simulink model "ThreePhasePVModule"  (R2025b)
settings: Solver=VariableStepAuto  StartTime=0.0  StopTime=1  RelTol=1e-3
undefined symbols (not defined in the file): Ppv
libraries: fl_lib x7, nesl_utility x5, simulink x1
settings Model: Creator=a6039  LastModifiedBy=agarcian
settings SolverCC: AlgebraicLoopSolver=TrustRegion
settings DebuggingCC: UnconnectedInputMsg=warning  UnconnectedOutputMsg=warning  UnconnectedLineMsg=warning
settings ModelReferenceCC: EnableRefExpFcnMdlSchedulingChecks=on
settings RTWCC: GPUComputeCapability=3.5  DLArmComputeVersion=19.05

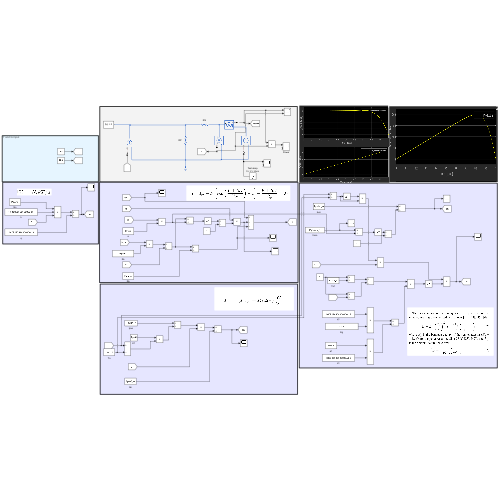
[thumbnail: Simulink's stored preview of the top-level diagram]
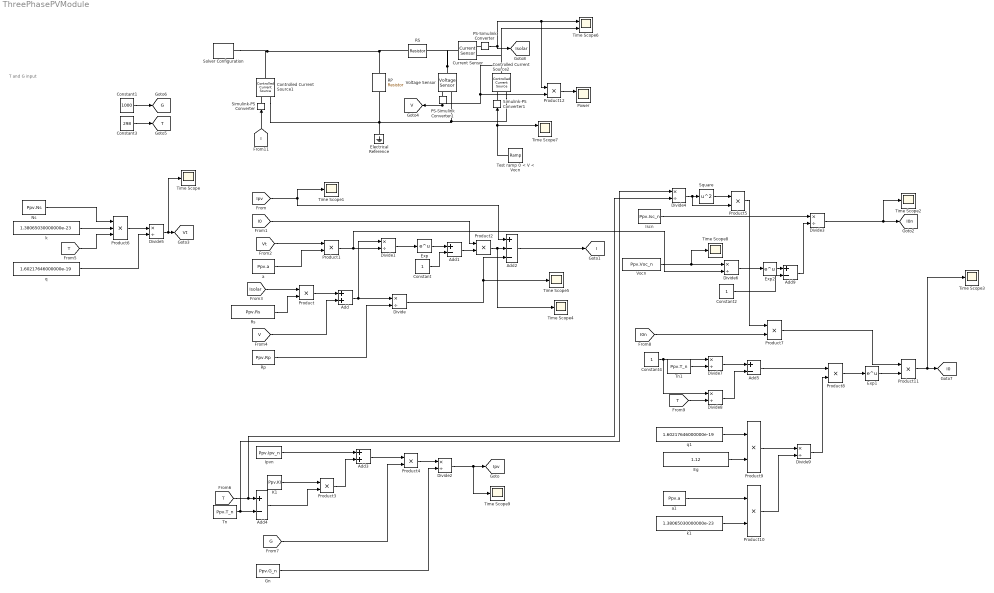
== system ThreePhasePVModule ==
  note: T and G input
  Add : Sum
  Add{1,4..5,9} (4 alike) : Sum  Inputs=+-
  Add2 : Sum  Inputs=+--
  Add3 : Sum
  Constant : Constant
  Constant1 : Constant  Value=1000
  Constant2 : Constant
  Constant3 : Constant  Value=298
  Constant4 : Constant
  Controlled Current Source1 : fl_lib/Electrical/Electrical Sources/Controlled Current Source
  Controlled Current Source2 : fl_lib/Electrical/Electrical Sources/Controlled Current Source
  Current Sensor : fl_lib/Electrical/Electrical Sensors/Current Sensor
  Divide{,1..9} (10 alike) : Product  Inputs=*/
  Eg : Constant  Value=1.12
  Electrical Reference : fl_lib/Electrical/Electrical Elements/Electrical Reference
  Exp : Math
  Exp1 : Math
  Exp2 : Math
  Gn : Constant  Value=Ppv.G_n
  Ipvn : Constant  Value=Ppv.Ipv_n
  Iscn : Constant  Value=Ppv.Isc_n
  K1 : Constant  Value=Ppv.KI
  Ns : Constant  Value=Ppv.Ns
  PS-Simulink Converter : nesl_utility/PS-Simulink Converter  PhysicalDomain=network_engine_domain  SubClassName=ps_output  LeftPortType=input  RightPortType=output  PseudoPeriodic=off  Frequencies=[]  VectorFormat=inherit  Unit=inherit  AffineConversion=off
  PS-Simulink Converter1 : nesl_utility/PS-Simulink Converter  PhysicalDomain=network_engine_domain  SubClassName=ps_output  LeftPortType=input  RightPortType=output  PseudoPeriodic=off  Frequencies=[]  VectorFormat=inherit  Unit=inherit  AffineConversion=off
  Power : Scope  NumInputPorts=2
      settings: TimeUnits=Metric (based on Time Span)  ActiveDisplayYMinimum=-158.2887  ActiveDisplayYMaximum=34.79764  YLabel=Amplitude  DataLoggingVariableName=ScopeData9
  Product{,1..5,7..12} (12 alike) : Product
  Product6 : Product  Inputs=3
  RP : fl_lib/Electrical/Electrical Elements/Resistor  R=Ppv.Rp Ohm  i_specify=off  i_priority=None  i=0 A  i_nominal_specify=off  i_nominal_value=1  i_nominal_unit=A  v_specify=off  v_priority=None  v=0 V  v_nominal_specify=off  v_nominal_value=1  v_nominal_unit=V
  RS : fl_lib/Electrical/Electrical Elements/Resistor  R=Ppv.Rs Ohm  i_specify=off  i_priority=None  i=0 A  i_nominal_specify=off  i_nominal_value=1  i_nominal_unit=A  v_specify=off  v_priority=None  v=0 V  v_nominal_specify=off  v_nominal_value=1  v_nominal_unit=V
  Rp : Constant  Value=Ppv.Rp
  Rs : Constant  Value=Ppv.Rs
  Simulink-PS Converter : nesl_utility/Simulink-PS Converter  PhysicalDomain=network_engine_domain  SubClassName=ps_input  LeftPortType=input  RightPortType=output  PseudoPeriodic=off  Frequencies=[]  NoiseDistribution=none  NoiseParameters=[]  Unit=1  AffineConversion=off  FilteringAndDerivatives=provide  SimscapeFilterOrder=1  InputFilterTimeConstant=0.001  UdotUserProvided=0
  Simulink-PS Converter1 : nesl_utility/Simulink-PS Converter  PhysicalDomain=network_engine_domain  SubClassName=ps_input  LeftPortType=input  RightPortType=output  PseudoPeriodic=off  Frequencies=[]  NoiseDistribution=none  NoiseParameters=[]  Unit=1  AffineConversion=off  FilteringAndDerivatives=provide  SimscapeFilterOrder=1  InputFilterTimeConstant=0.001  UdotUserProvided=0
  Solver Configuration : nesl_utility/Solver Configuration  PhysicalDomain=network_engine_domain  SubClassName=solver  LeftPortType=input  RightPortType=generic  Tones=[]  Harmonics=[]  SimulateNoise=off  Profile=off  UseLocalSampling=off  EnableSwitchedLinearOptims=on  FrequencyDomain=off  UseCCode=off  RelTol=0.001  AbsTol=0.001  MinStep=1e-09  ToWorkspace=off  RevertToSquareIcSolve=off  NumHomotopyIterations=100  PhasorMode=off  PhasorModeNumHarmonics=1  ConsistencySolver=NEWTON_XTOL_AFTER_FTOL  IndexReductionMethod=DerivativeReplacement  DoDC=off  ResidualTolerance=1e-09  ConsistencyTolSource=GLOBAL  ConsistencyAbsTol=0.001  ConsistencyRelTol=0.001  ConsistencyTolFactor=0.001  UseLocalSolver=off  LocalSolverChoice=NE_BACKWARD_EULER_ADVANCER  ResolveIndetEquations=on  FunctionEvalNumThread=1  LocalSolverSampleTime=0.001  DoFixedCost=off  MaxNonlinIter=3  MaxModeIter=2  ComputeImpulses=off  ImpulseIterations=2  LinearAlgebra=auto  LinearAlgebraNumThread=0  EquationFormulation=NE_TIME_EF  DelaysMemoryBudget=1024  AutomaticFiltering=on  FilteringTimeConstant=0.001  PartitionStorageMethod=AS_NEEDED  PartitionMemoryBudget=1024  PartitionMethod=ROBUST  MultibodyUseLocalSolver=off  MultibodyLocalSolverChoice=ODE1  MultibodyLocalSolverSampleTime=0.001
  Square : Math  Operator=square
  Test ramp 0 < V < Vocn : simulink/Sources/Ramp  slope=Ppv.Voc_n  start=0  InitialOutput=0
  Time Scope{,1..5,8..9} (8 alike) : Scope
      Time Scope settings: TimeUnits=Metric (based on Time Span)  ActiveDisplayYMinimum=0.3867  ActiveDisplayYMaximum=2.3867  YLabel=Amplitude  DataLoggingVariableName=ScopeData2
      Time Scope1 settings: TimeUnits=Metric (based on Time Span)  ActiveDisplayYMinimum=7.21  ActiveDisplayYMaximum=9.21  YLabel=Amplitude  DataLoggingVariableName=ScopeData3
      Time Scope2 settings: TimeUnits=Metric (based on Time Span)  ActiveDisplayYMinimum=8.7E-8  ActiveDisplayYMaximum=1.07E-7  YLabel=Amplitude
      Time Scope3 settings: TimeUnits=Metric (based on Time Span)  ActiveDisplayYMinimum=8.7E-8  ActiveDisplayYMaximum=1.07E-7  YLabel=Amplitude  DataLoggingVariableName=ScopeData4
      Time Scope4 settings: TimeUnits=Metric (based on Time Span)  ActiveDisplayYMinimum=-1.01635  ActiveDisplayYMaximum=9.14713  YLabel=Amplitude  DataLoggingVariableName=ScopeData5
      Time Scope5 settings: TimeUnits=Metric (based on Time Span)  ActiveDisplayYMinimum=-0.00499  ActiveDisplayYMaximum=0.08851  YLabel=Amplitude  DataLoggingVariableName=ScopeData6
      Time Scope8 settings: TimeUnits=Metric (based on Time Span)  ActiveDisplayYMinimum=776.6  ActiveDisplayYMaximum=2776.6  YLabel=Amplitude  DataLoggingVariableName=ScopeData8
      Time Scope9 settings: TimeUnits=Metric (based on Time Span)  ActiveDisplayYMinimum=7.21  ActiveDisplayYMaximum=9.21  YLabel=Amplitude
  Time Scope6 : Scope  NumInputPorts=2
      settings: TimeUnits=Metric (based on Time Span)  ActiveDisplayYMinimum=-1.1133  ActiveDisplayYMaximum=9.23623  YLabel=Amplitude  DataLoggingVariableName=ScopeData7
  Time Scope7 : Scope  NumInputPorts=2
      settings: TimeUnits=Metric (based on Time Span)  ActiveDisplayYMinimum=-4.1125  ActiveDisplayYMaximum=37.0125  YLabel=Amplitude
  Tn : Constant  Value=Ppv.T_n
  Tn1 : Constant  Value=Ppv.T_n
  Vocn : Constant  Value=Ppv.Voc_n
  Voltage Sensor : fl_lib/Electrical/Electrical Sensors/Voltage Sensor
  a : Constant  Value=Ppv.a
  a1 : Constant  Value=Ppv.a
  k : Constant  Value=1.38065030000000e-23
  k1 : Constant  Value=1.38065030000000e-23
  q : Constant  Value=1.60217646000000e-19
  q1 : Constant  Value=1.60217646000000e-19
  tag scope: G=global, I0=global, I0n=global, I=global, Ipv=global, Isolar=global, T=global, V=global, Vt=global
  wires:
  [Isolar] -> Product/1
  Rs/1 -> Product/2
  Product/1 -> Add/1
  [V] -> Add/2
  Add/1 -> Divide1/1, Divide/1
  Rp/1 -> Divide/2
  [Vt] -> Product1/1
  a/1 -> Product1/2
  Product1/1 -> Divide6/2, Divide1/2
  Divide1/1 -> Exp/1
  Exp/1 -> Add1/1
  Constant/1 -> Add1/2
  Add1/1 -> Product2/2
  [I0] -> Product2/1
  Product2/1 -> Time Scope4/1, Add2/2
  Divide/1 -> Time Scope5/1, Add2/3
  K1/1 -> Product3/1
  Add4/1 -> Product3/2
  Ipvn/1 -> Add3/1
  Product3/1 -> Add3/2
  Add3/1 -> Product4/1
  [G] -> Product4/2
  Product4/1 -> Divide2/1
  Gn/1 -> Divide2/2
  Divide2/1 -> Time Scope9/1, [Ipv]
  Add2/1 -> [I]
  Constant2/1 -> Add9/2
  Divide3/1 -> Time Scope2/1, [I0n]
  k/1 -> Product6/2
  [T] -> Product6/3
  Product6/1 -> Divide5/1
  q/1 -> Divide5/2
  Divide5/1 -> Time Scope/1, [Vt]
  PS-Simulink Converter1/1 -> Time Scope6/2, Product12/2, [V]
  Constant1/1 -> [G]
  Constant3/1 -> [T]
  [T] -> Divide4/2, Add4/1
  Tn/1 -> Divide4/1, Add4/2
  Iscn/1 -> Divide3/1
  Vocn/1 -> Time Scope8/1, Divide6/1
  Divide6/1 -> Exp2/1
  Exp2/1 -> Add9/1
  Add9/1 -> Divide3/2
  Divide4/1 -> Product5/2, Square/1
  Square/1 -> Product5/1
  [I0n] -> Product7/2
  Product5/1 -> Product7/1
  Constant4/1 -> Divide8/1, Divide7/1
  Tn1/1 -> Divide7/2
  Divide7/1 -> Add5/1
  [T] -> Divide8/2
  Divide8/1 -> Add5/2
  Add5/1 -> Product8/1
  q1/1 -> Product9/1
  Eg/1 -> Product9/2
  Product9/1 -> Divide9/1
  a1/1 -> Product10/1
  k1/1 -> Product10/2
  Product10/1 -> Divide9/2
  Divide9/1 -> Product8/2
  Product8/1 -> Exp1/1
  Exp1/1 -> Product11/2
  Product7/1 -> Product11/1
  Product11/1 -> Time Scope3/1, [I0]
  Test ramp 0 < V < Vocn/1 -> Time Scope7/1, Simulink-PS Converter1/1
  PS-Simulink Converter/1 -> [Isolar], Product12/1, Time Scope6/1
  [Ipv] -> Add2/1, Time Scope1/1
  Ns/1 -> Product6/1
  Product12/1 -> Power/1
  [I] -> Simulink-PS Converter/1
  connections:
  Controlled Current Source1/RConn2 -- Electrical Reference/LConn1 -- Controlled Current Source2/RConn2 -- Voltage Sensor/RConn2 -- RP/RConn1
  Controlled Current Source1/LConn1 -- Solver Configuration/RConn1 -- RS/RConn1 -- RP/LConn1
  Voltage Sensor/LConn1 -- RS/LConn1 -- Current Sensor/LConn1
  Simulink-PS Converter/RConn1 -- Controlled Current Source1/RConn1
  PS-Simulink Converter1/LConn1 -- Voltage Sensor/RConn1
  PS-Simulink Converter/LConn1 -- Current Sensor/RConn1
  Controlled Current Source2/LConn1 -- Current Sensor/RConn2
  Simulink-PS Converter1/RConn1 -- Controlled Current Source2/RConn1
